simulink model "LQR"  (R2023a)
settings: Solver=VariableStepAuto  StartTime=0.0  StopTime=30  RelTol=1e-3
undefined symbols (not defined in the file or in its folder): Continuous, Time
libraries: ctrlSharedLib x2
settings Model: Creator=BRL  LastModifiedBy=BRL

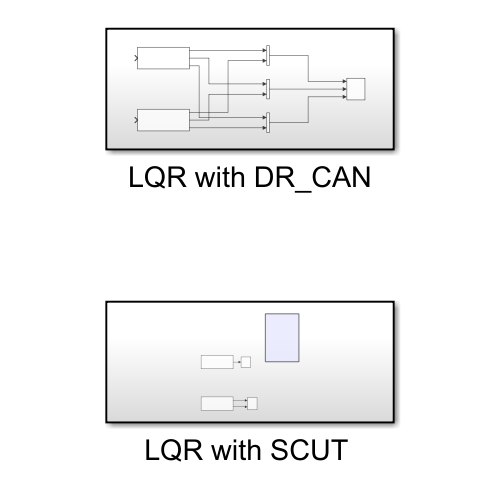
[thumbnail: Simulink's stored preview of the top-level diagram]
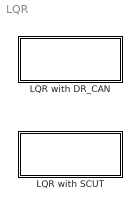
== system LQR ==
  LQR with DR_CAN : Subsystem
  "LQR with SCUT " : Subsystem

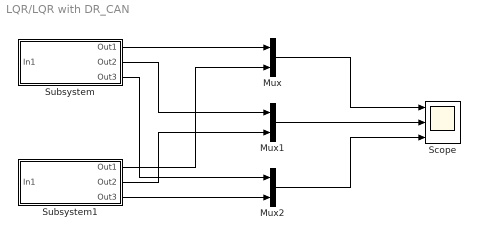
== system LQR/LQR with DR_CAN ==
  Mux : Mux  Inputs=2
  Mux1 : Mux  Inputs=2
  Mux2 : Mux  Inputs=2
  Scope : Scope  NumInputPorts=3
  Subsystem : Subsystem
  Subsystem1 : Subsystem
  wires:
  Subsystem1/2(Out2) -> Mux1/2
  Subsystem1/1(Out1) -> Mux/2
  Subsystem/1(Out1) -> Mux/1
  Mux/1 -> Scope/1
  Subsystem1/3(Out3) -> Mux2/2
  Mux2/1 -> Scope/3
  Subsystem/3(Out3) -> Mux2/1
  Subsystem/2(Out2) -> Mux1/1
  Mux1/1 -> Scope/2

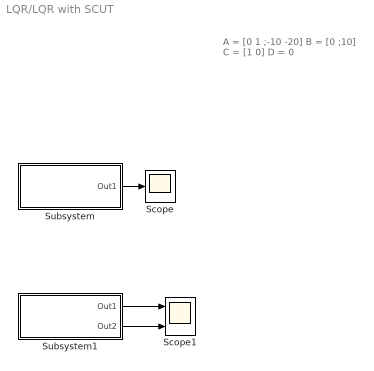
== system LQR/LQR with SCUT  ==
  note: A = [0 1 ;-10 -20]
      | B = [0 ;10]
      | C = [1 0]
      | D = 0
  Scope : Scope
  Scope1 : Scope  NumInputPorts=2
  Subsystem : Subsystem
  Subsystem1 : Subsystem
  wires:
  Subsystem/1(Out1) -> Scope/1
  Subsystem1/1(Out1) -> Scope1/1
  Subsystem1/2(Out2) -> Scope1/2

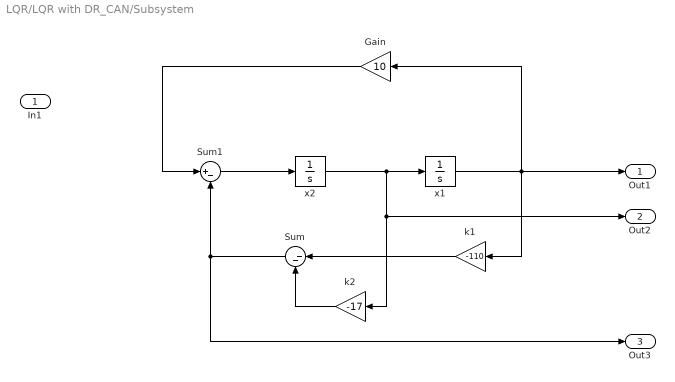
== system LQR/LQR with DR_CAN/Subsystem ==
  In1 : Inport
  Gain : Gain  Gain=10
  Sum : Sum  Inputs=|--
  Sum1 : Sum  Inputs=|+-
  k1 : Gain  Gain=-110
  k2 : Gain  Gain=-17
  x1 : Integrator  InitialCondition=5
  x2 : Integrator
  Out1 : Outport
  Out2 : Outport  Port=2
  Out3 : Outport  Port=3
  wires:
  k2/1 -> Sum/2
  x2/1 -> Out2/1, k2/1, x1/1
  Sum/1 -> Out3/1, Sum1/2
  Gain/1 -> Sum1/1
  x1/1 -> k1/1, Out1/1, Gain/1
  k1/1 -> Sum/1
  Sum1/1 -> x2/1

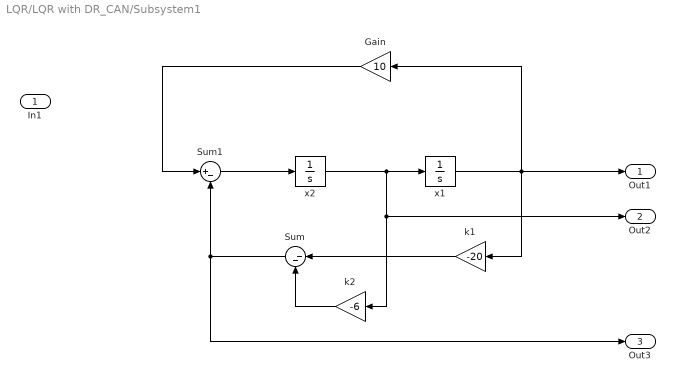
== system LQR/LQR with DR_CAN/Subsystem1 ==
  In1 : Inport
  Gain : Gain  Gain=10
  Sum : Sum  Inputs=|--
  Sum1 : Sum  Inputs=|+-
  k1 : Gain  Gain=-20
  k2 : Gain  Gain=-6
  x1 : Integrator  InitialCondition=5
  x2 : Integrator
  Out1 : Outport
  Out2 : Outport  Port=2
  Out3 : Outport  Port=3
  wires:
  k2/1 -> Sum/2
  x2/1 -> Out2/1, k2/1, x1/1
  Sum/1 -> Out3/1, Sum1/2
  Gain/1 -> Sum1/1
  x1/1 -> k1/1, Out1/1, Gain/1
  k1/1 -> Sum/1
  Sum1/1 -> x2/1

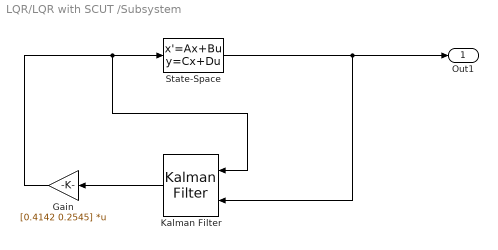
== system LQR/LQR with SCUT /Subsystem ==
  Gain : Gain  Gain=[0.4142 0.2545]  Multiplication=Matrix(K*u)
  Kalman Filter : ctrlSharedLib/Kalman Filter  TimeDomain=Continuous-Time  UseCurrentEstimator=on  ModelSource=Individual A, B, C, D matrices  ModelSourceVariable=ss(0.95,1,1,0,1)  A=[0 1 ;-10 -20]  B=[0 ;10]  C=[1 0]  D=0  NumberOfStates=1  NumberOfInputs=1  NumberOfOutputs=1  InitialEstimateSource=Dialog  X0=0  P0=10  UseK=off  UseGH=off  NumberOfProcessNoiseInputs=1  G=1  TimeInvariantG=on  H=0  TimeInvariantH=on  Q=0.05  TimeInvariantQ=on  R=1  TimeInvariantR=on  N=0  TimeInvariantN=on  AddInputPort=on  AddEnablePort=off  OutputEstimatedY=off  OutputP=off  Ts=-1
  State-Space : StateSpace  A=[0 1; -10 -20]  B=[0; 10]  C=[1 0]  D=0  InitialCondition=1
  Out1 : Outport
  wires:
  Gain/1 -> Kalman Filter/1, State-Space/1
  State-Space/1 -> Out1/1, Kalman Filter/2
  Kalman Filter/1 -> Gain/1

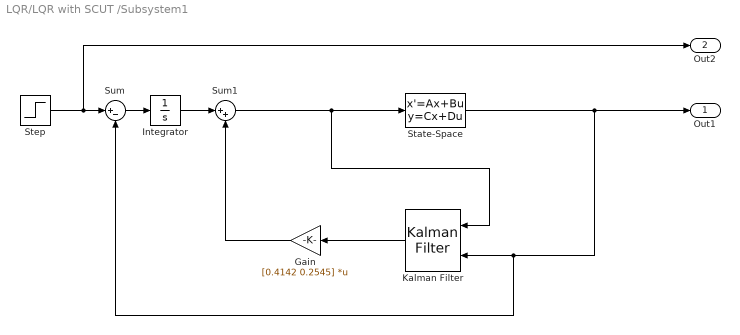
== system LQR/LQR with SCUT /Subsystem1 ==
  Gain : Gain  Gain=[0.4142 0.2545]  Multiplication=Matrix(K*u)
  Integrator : Integrator
  Kalman Filter : ctrlSharedLib/Kalman Filter  TimeDomain=Continuous-Time  UseCurrentEstimator=on  ModelSource=Individual A, B, C, D matrices  ModelSourceVariable=ss(0.95,1,1,0,1)  A=[0 1 ;-10 -20]  B=[0 ;10]  C=[1 0]  D=0  NumberOfStates=1  NumberOfInputs=1  NumberOfOutputs=1  InitialEstimateSource=Dialog  X0=0  P0=10  UseK=off  UseGH=off  NumberOfProcessNoiseInputs=1  G=1  TimeInvariantG=on  H=0  TimeInvariantH=on  Q=0.05  TimeInvariantQ=on  R=1  TimeInvariantR=on  N=0  TimeInvariantN=on  AddInputPort=on  AddEnablePort=off  OutputEstimatedY=off  OutputP=off  Ts=-1
  State-Space : StateSpace  A=[0 1; -10 -20]  B=[0; 10]  C=[1 0]  D=0  InitialCondition=0
  Step : Step  SampleTime=0
  Sum : Sum  Inputs=|+-
  Sum1 : Sum  Inputs=|++
  Out1 : Outport
  Out2 : Outport  Port=2
  wires:
  Gain/1 -> Sum1/2
  State-Space/1 -> Out1/1, Kalman Filter/2, Sum/2
  Kalman Filter/1 -> Gain/1
  Step/1 -> Out2/1, Sum/1
  Sum1/1 -> Kalman Filter/1, State-Space/1
  Sum/1 -> Integrator/1
  Integrator/1 -> Sum1/1
